simulink model "CS4"  (R2023b)
settings: Solver=VariableStepAuto  StartTime=0.0  StopTime=0.05  RelTol=1e-3
undefined symbols (not defined in the file): Angle, Magnitude
libraries: spsCurrentMeasurementLib x3, spsSeriesRLCBranchLib x2, spsLinearTransformerLib x2, spsACVoltageSourceLib x1, spsVoltageMeasurementLib x1, spspowerguiLib x1
settings Model: Creator=gupta  LastModifiedBy=gupta
settings RTWCC: GPUComputeCapability=5.0

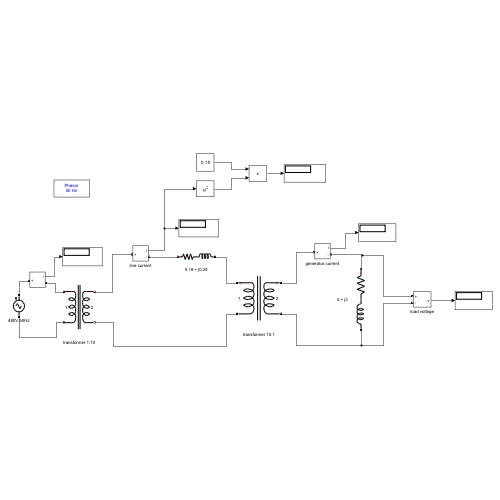
[thumbnail: Simulink's stored preview of the top-level diagram]
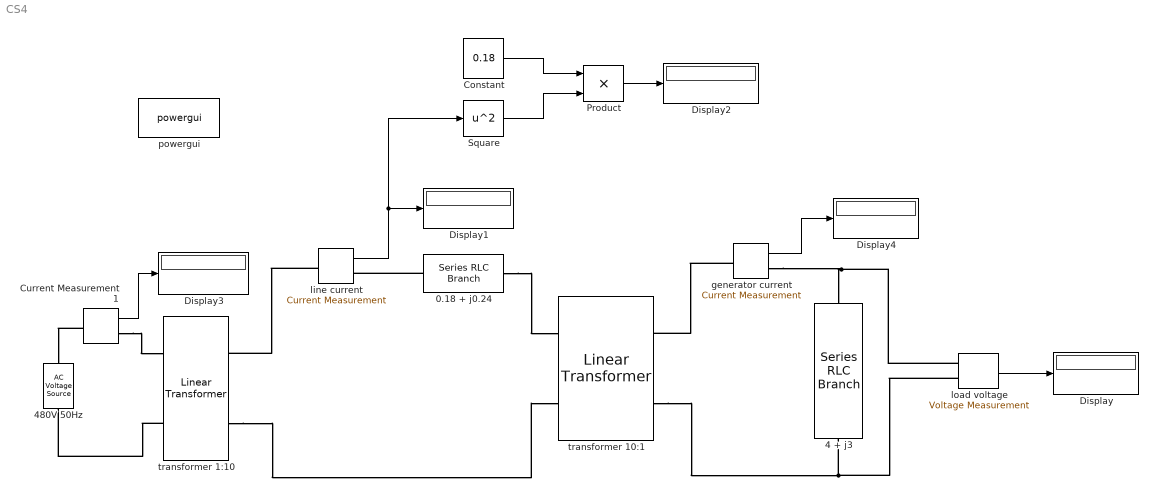
== system CS4 ==
  0.18 + j0.24 : spsSeriesRLCBranchLib/Series RLC Branch  LConnTagsString=__new0  RConnTagsString=__new0  BranchType=RL  Resistance=0.18  Inductance=0.0007639  SetiL0=off  InitialCurrent=0  Capacitance=1e-6  Setx0=off  InitialVoltage=0  Measurements=None
  4 + j3 : spsSeriesRLCBranchLib/Series RLC Branch  LConnTagsString=__new0  RConnTagsString=__new0  BranchType=RL  Resistance=4  Inductance=0.009549  SetiL0=off  InitialCurrent=0  Capacitance=1e-6  Setx0=off  InitialVoltage=0  Measurements=None
  480V 50Hz : spsACVoltageSourceLib/AC Voltage Source  Amplitude=480  Phase=0  Frequency=50  SampleTime=0  Measurements=None  BusType=swing  Pref=10e3  Qref=0  Qmin=-inf  Qmax=+inf
  Constant : Constant  Value=0.18
  Current Measurement1 : spsCurrentMeasurementLib/Current Measurement  PhasorSimulation=on  OutputType=Magnitude-Angle  PSBequivalent=0
  Display{,1..4} (5 alike) : Display
  Product : Product
  Square : Math  Operator=square
  generator current : spsCurrentMeasurementLib/Current Measurement  PhasorSimulation=on  OutputType=Magnitude-Angle  PSBequivalent=0
  line current : spsCurrentMeasurementLib/Current Measurement  PhasorSimulation=on  OutputType=Magnitude-Angle  PSBequivalent=0
  load voltage : spsVoltageMeasurementLib/Voltage Measurement  PhasorSimulation=on  OutputType=Magnitude-Angle  PSBequivalent=0
  powergui : spspowerguiLib/powergui  Priority=1  SimulationMode=Phasor  SampleTime=50e-6  frequency=50  Iterations=50  frequencyindice=50  Pbase=100e6  ErrMax=1e-4  UnitsV=kV  UnitsW=MW  buscounter=0  FunctionMessages=off  echomessages=off  EnableUseOfTLC=off  CurrentSourceSwitches=off  DisableSnubberDevices=off  DisableRonSwitches=off  DisableVfSwitches=off  DisplayEquations=off  AutomaticDiscreteSolvers=off  SolverType=Tustin/Backward Euler (TBE)  Interpol=off  ExternalGateDelay=off  methode=off  Ts=100  x0status=blocks  SPID=on  SwTol=0  HookPort=off  NonlinearTolerance=1e-4  nMaxIteration=100  ContinueOnMaxIteration=off  RestoreLinks=warning  ResistiveCurrentMeasurement=off  Frange=[0:2:500]  Ylog=off  Xlog=on  ShowGrid=off  save=off  variable=ZData  structure=0  ZoomFFT=off  StartTime=0.0  cycles=1  DisplayStyle=1  fundamental=60  FreqAxis=off  MaxFrequency=1000  frequencyindicesteady=1  RmsSteady=1  display=off
  transformer 10:1 : spsLinearTransformerLib/Linear Transformer  UNITS=SI  NominalPower=[ 250e6 50 ]  winding1=[4800 0.000000001 0.000000001]  winding2=[480 0.000000001 0.000000001]  ThreeWindings=off  winding3=[3.15e+05 0.7938 0.10107]  RmLm=[1.0804e+06 3439.2]  Measurements=None  DataType=on
  transformer 1:10 : spsLinearTransformerLib/Linear Transformer  UNITS=SI  NominalPower=[ 250e6 50 ]  winding1=[480 0.000000001 0.000000001]  winding2=[4800 0.000000001 0.000000001]  ThreeWindings=off  winding3=[3.15e+05 0.7938 0.10107]  RmLm=[1.0804e+06 3439.2]  Measurements=None  DataType=on
  wires:
  load voltage/1 -> Display/1
  line current/1 -> Square/1, Display1/1
  Constant/1 -> Product/1
  Square/1 -> Product/2
  Product/1 -> Display2/1
  Current Measurement1/1 -> Display3/1
  generator current/1 -> Display4/1
  connections:
  0.18 + j0.24/LConn1 -- line current/RConn1
  load voltage/LConn1 -- generator current/RConn1 -- 4 + j3/LConn1
  load voltage/LConn2 -- transformer 10:1/RConn2 -- 4 + j3/RConn1
  Current Measurement1/RConn1 -- transformer 1:10/LConn1
  Current Measurement1/LConn1 -- 480V 50Hz/RConn1
  transformer 1:10/LConn2 -- 480V 50Hz/LConn1
  line current/LConn1 -- transformer 1:10/RConn1
  0.18 + j0.24/RConn1 -- transformer 10:1/LConn1
  transformer 1:10/RConn2 -- transformer 10:1/LConn2
  generator current/LConn1 -- transformer 10:1/RConn1
